simulink model "Sample155"  (Simulink 7.6)
settings: Solver=ode45  StartTime=0.0  StopTime=10.0  MaxStep=0.2  RelTol=1e-3
undefined symbols (not defined in the file): randint
libraries: commrandsrc2 x1, commdigbbndcpm2 x1, commdigbbndfm2 x1, dspsrcs4 x1, commblkcod2 x1
settings Model: Creator=Administrator  LastModifiedBy=zhangling
settings DataIOCC: ExternalInput=A

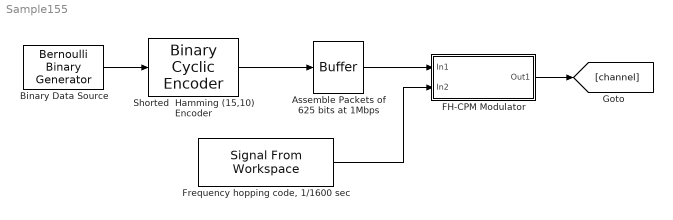
== system Sample155 ==
  Assemble Packets of 625 bits at 1Mbps : Buffer  N=625  TreatMby1Signals=One channel
  Binary Data Source : commrandsrc2/Bernoulli Binary Generator  DialogController=commDDGCreate  DialogControllerArgs=DataTag0  SystemSampleTime=-1  P=[.5]  seed=[12345]  Ts=1.5e-6  frameBased=on  sampPerFrame=10  orient=off  outDataType=double
  FH-CPM Modulator : Subsystem
  "Frequency hopping code, 1/1600 sec " : dspsrcs4/Signal From Workspace  SystemSampleTime=-1  X=randint(1,100,78)  Ts=1/1600  nsamps=1  OutputAfterFinalValue=Cyclic repetition  ignoreOrWarnInputAndFrameLengths=off
  Shorted  Hamming (15,10) Encoder : commblkcod2/Binary Cyclic Encoder  SystemSampleTime=-1  n=15  p=[1 1 0 1 0 1]
  wires:
  Binary Data Source/1 -> Shorted  Hamming (15,10) Encoder/1
  Shorted  Hamming (15,10) Encoder/1 -> Assemble Packets of 625 bits at 1Mbps/1
  Assemble Packets of 625 bits at 1Mbps/1 -> FH-CPM Modulator/1(In1)
  FH-CPM Modulator/1(Out1) -> [channel]
  "Frequency hopping code, 1/1600 sec "/1 -> FH-CPM Modulator/2(In2)

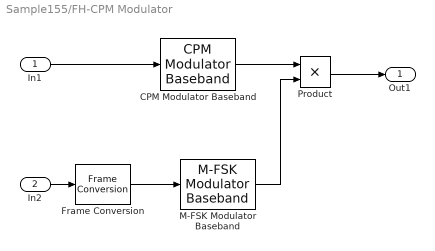
== system Sample155/FH-CPM Modulator ==
  In1 : Inport
  In2 : Inport  Port=2
  CPM Modulator Baseband : commdigbbndcpm2/CPM Modulator Baseband  Mnum=2  inputType=Bit  mappingType=Binary  modIdx=0.3  pulseShape=Gaussian  BT=0.5  mainLobePulseLength=1  rollOff=0.2  pulseLength=1  preHistory=1  phaseOffset=0  samplesPerSymbol=8  RateOptions=Enforce single-rate processing  outDataType=double
  Frame Conversion : FrameConversion
  M-FSK Modulator Baseband : commdigbbndfm2/M-FSK Modulator Baseband  M=79  InType=Integer  Enc=Binary  freqSep=1e6  phaseType=Continuous  numSamp=6.25e4  RateOptions=Enforce single-rate processing  outDataType=double
  Product : Product  RndMeth=Zero
  Out1 : Outport
  wires:
  In1/1 -> CPM Modulator Baseband/1
  CPM Modulator Baseband/1 -> Product/1
  Product/1 -> Out1/1
  M-FSK Modulator Baseband/1 -> Product/2
  In2/1 -> Frame Conversion/1
  Frame Conversion/1 -> M-FSK Modulator Baseband/1
